simulink model "kenar_belirleme"  (R2013b)
settings: Solver=FixedStepDiscrete  StartTime=0.0  StopTime=inf  RelTol=1e-3
undefined symbols (not defined in the file or in its folder): IsPositionTracked, IsSkeletonTracked, JointDepthIndices, JointImageIndices, JointTrackingState, JointWorldCoordinates, none, PositionDepthIndices, PositionImageIndices, PositionWorldCoordinates, SegmentationData, SkeletonTrackingID, videoinput
libraries: visionsinks x3, visiontextngfix x1, visionanalysis x1, imaqlib x1
settings Model: FPTRunName=Active  ExtModeAutoUpdateStatusClock=off  Creator=The MathWorks Inc.  LastModifiedBy=Zeynep
settings DataIOCC: LimitDataPoints=off  SignalLoggingSaveFormat=ModelDataLogs  SaveOutput=off  SaveTime=off  SignalLoggingName=sigsOut
settings OptimizationCC: ExpressionDepthLimit=2147483647  InitFltsAndDblsToZero=on
settings DebuggingCC: CheckExecutionContextPreStartOutputMsg=on  CheckExecutionContextRuntimeOutputMsg=on  SignalResolutionControl=TryResolveAllWithWarning  SolverPrmCheckMsg=none  MultiTaskDSMMsg=warning  MultiTaskCondExecSysMsg=none  SigSpecEnsureSampleTimeMsg=none  FcnCallInpInsideContextMsg=UseLocalSettings  StateNameClashWarn=warning
settings HardwareCC: TargetLongLongMode=on  TargetEndianess=LittleEndian  TargetHWDeviceType=Generic->MATLAB Host Computer  ProdEqTarget=off
settings RTWCC: IncludeERTFirstTime=on
settings GRTTargetCC: TargetFcnLib=ansi_tfl_tmw_new.mat  CombineOutputUpdateFcns=off  GRTInterface=on

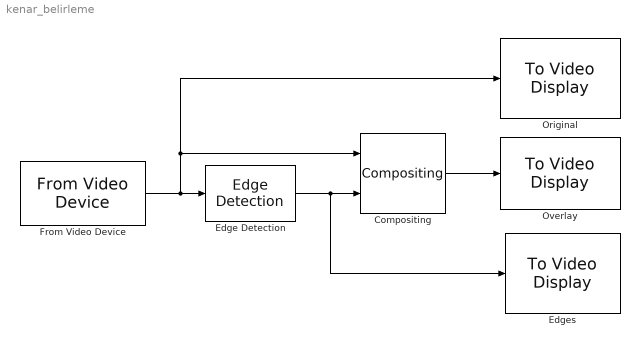
== system kenar_belirleme ==
  Compositing : visiontextngfix/Compositing  operation=Highlight selected pixels  bFacSrc=Input port  mFacSrc=Input port  bFactor=0.75  mFactor=1  source=Specify via dialog  coordinates=[1 1]  prodOutputMode=Binary point scaling  prodOutputWordLength=32  prodOutputFracLength=10  roundingMode=Floor  overflowMode=off
  Edge Detection : visionanalysis/Edge Detection  method=Prewitt  outputType=Binary image  userDefinedThreshold=on  thresholdSource=Specify via dialog  threshold=single(15/256)  thresholdTuning=4  edgeThinning=on  threshold_canny=[0.25 0.60]  autoPercent=70  sigma=1  roundingMode=Floor  overflowMode=off
  Edges : visionsinks/To Video Display  inputType=Intensity  imagePorts=Separate color signals  OutputDevice=On-screen video monitor  fullScreen=off  videoWindowX=222  videoWindowY=583  saveWindowSize=off  videoWindowWidth=1280  videoWindowHeight=720  dataOrg=Column-major  openAtMdlStart=on  isWindowOpen=off  inputColorFormat=RGB
  From Video Device : imaqlib/From Video Device  DeviceMenu=winvideo 1 (USB2.0 UVC HD Webcam)  Device=winvideo 1 (USB2.0 UVC HD Webcam)  ObjConstructor=videoinput('winvideo', 1)  VideoFormatMenu=MJPG_1280x720  VideoFormat=MJPG_1280x720  VideoSource=input1  ROIPosition=[0 0 720 1280]  EnableHWTrigger=off  TriggerConfiguration=none/none  SampleTime=1/30  OutputPortsMode=One multidimensional signal  DataType=single  CanDoHWTrigger=no  ReturnedColorSpace=grayscale  BlockHandle=30.1971  ROIWidth=1280  ROIHeight=720  ROIColumn=0  ROIRow=0  EngXMLPath=C:\Program Files\MATLAB\R2013b\toolbox\imaq\imaq\private  DevXMLPath=C:\Program Files\MATLAB\R2013b\toolbox\imaq\imaqadaptors\win64  EngLibPath=C:\Program Files\MATLAB\R2013b\toolbox\imaq\imaqblks\imaqmex\win64  ColorSpace=grayscale  BayerSensorAlignment=grbg  AllMetadata=IsPositionTracked;IsSkeletonTracked;JointDepthIndices;JointImageIndices;JointTrackingState;JointWorldCoordinates;PositionDepthIndices;PositionImageIndices;PositionWorldCoordinates;SegmentationData;SkeletonTrackingID
  Original : visionsinks/To Video Display  inputType=Intensity  imagePorts=Separate color signals  OutputDevice=On-screen video monitor  fullScreen=off  videoWindowX=42  videoWindowY=115  saveWindowSize=off  videoWindowWidth=1280  videoWindowHeight=720  dataOrg=Column-major  openAtMdlStart=on  isWindowOpen=off  inputColorFormat=RGB
  Overlay : visionsinks/To Video Display  inputType=Intensity  imagePorts=Separate color signals  OutputDevice=On-screen video monitor  fullScreen=off  videoWindowX=380  videoWindowY=70  saveWindowSize=off  videoWindowWidth=1280  videoWindowHeight=720  dataOrg=Column-major  openAtMdlStart=on  isWindowOpen=off  inputColorFormat=RGB
  wires:
  From Video Device/1 -> Edge Detection/1, Original/1, Compositing/1
  Compositing/1 -> Overlay/1
  Edge Detection/1 -> Edges/1, Compositing/2
